simulink model "CS_PIDPr"  (R2014b)
settings: Solver=ode5  StartTime=0.0  StopTime=Te  FixedStep=Tm  RelTol=1e-3
StopFcn:
  | %salida(simout)
values from neighbouring files (symbols this model uses):
  D = 0    [globales.mat]
  I = 0    [globales.mat]
  Kb = 0    [globales.mat]
  P = 0.1    [globales.mat]
  Pf = 50    [globales.mat]
  Pi = -50    [globales.mat]
  Tm = 0.5    [globales.mat]
  Tp = 5    [globales.mat]
undefined symbols (not defined in the file or in its folder): A, B
undefined symbols (not defined in the file): Fcd, Fcp, Np
settings Model: ExtModeTrigDuration=100000  Creator=Equipo-Servo  LastModifiedBy=E. Rubio
settings DebuggingCC: UnderspecifiedInitializationDetection=Classic  MergeDetectMultiDrivingBlocksExec=none  StateNameClashWarn=warning
settings HardwareCC: ProdIntDivRoundTo=Zero  ProdEndianess=LittleEndian  ProdHWDeviceType=Generic->32-bit x86 compatible
settings RTWCC: SystemTargetFile=rtwin.tlc  TemplateMakefile=rtwin.tmf  Description=Real-Time Windows Target  ProcessScript=rtwin_make_rtw_hook  RTWCompilerOptimization=On
settings CodeAppCC: MaxIdLength=95
settings RTWinTargetCC: TargetLibSuffix=_rtwin.lib  TargetPreCompLibLocation=C:\Program Files\MATLAB\R2014b\toolbox\rtw\targets\rtwin\lib\win64

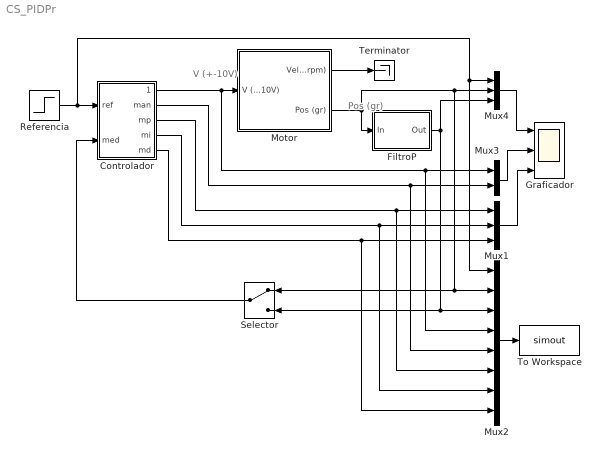
== system CS_PIDPr ==
  note: Pos
      | (gr)
  note: V (+-10V)
  Controlador : Subsystem  mask{T=Tm, P=P, I=I, Kb=Kb, D=D, Fcd=Fcd}
      mask prompts: T "Período de muestreo"; Kb "Kb (anti windup)"; Fcd "Fcd (Hz)"
      mask init:
      | N = 2*pi*Fcd;
  FiltroP : Subsystem  mask{N=Np, Fc=Fcp, Fm=1/Tm}
      mask prompts: N "Orden del filtro (Butterworth)"; Fc "Frecuencia de corte (Fc<Fm/2)"; Fm "Frecuencia de muestreo"
      mask init:
      | Fn = Fm/2;   % Frecuencia de Nyquist
      | [B,A] = butter(N,Fc/Fn);
  Graficador : Scope  NumInputPorts=3
      settings: TimeRange=10  YMin=-100~-15~-15  YMax=150~15~10  SampleTime=Tm
  Motor : Subsystem
  Mux1 : Mux  Inputs=3
  Mux2 : Mux  Inputs=8
  Mux3 : Mux  Inputs=2
  Mux4 : Mux  Inputs=3
  Referencia : Step  Time=Tp  Before=Pi  After=Pf  SampleTime=0
  Selector : ManualSwitch
  Terminator : Terminator
  To Workspace : ToWorkspace  VariableName=simout  SaveFormat=Structure With Time  SampleTime=Tm
  wires:
  Mux4/1 -> Graficador/1
  Motor/2(Pos (gr)) -> FiltroP/1(In), Selector/1, Mux2/2, Mux4/2
  Referencia/1 -> Mux2/1, Mux4/1, Controlador/1(ref)
  Mux2/1 -> To Workspace/1
  Controlador/1(mans) -> Motor/1(V (+-10V)), Mux2/4, Mux3/1
  FiltroP/1(Out) -> Selector/2, Mux2/3, Mux4/3
  Controlador/2(man) -> Mux2/5, Mux3/2
  Controlador/3(mp) -> Mux1/1, Mux2/6
  Controlador/4(mi) -> Mux2/7, Mux1/2
  Controlador/5(md) -> Mux2/8, Mux1/3
  Selector/1 -> Controlador/2(med)
  Mux3/1 -> Graficador/2
  Mux1/1 -> Graficador/3
  Motor/1(Vel (rpm)) -> Terminator/1

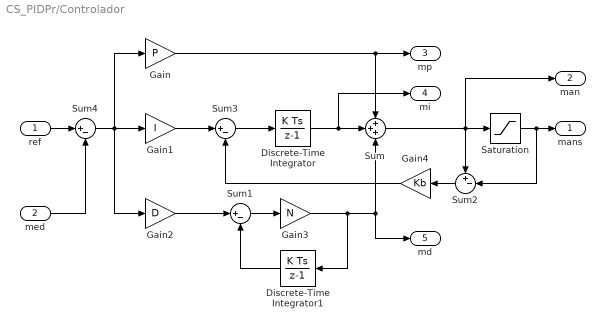
== system CS_PIDPr/Controlador ==
  ref : Inport
  med : Inport  Port=2
  Discrete-Time Integrator : DiscreteIntegrator  SampleTime=T
  Discrete-Time Integrator1 : DiscreteIntegrator  SampleTime=T
  Gain : Gain  Gain=P
  Gain1 : Gain  Gain=I
  Gain2 : Gain  Gain=D
  Gain3 : Gain  Gain=N
  Gain4 : Gain  Gain=Kb
  Saturation : Saturate  UpperLimit=10  LowerLimit=-10
  Sum : Sum  Inputs=+++
  Sum1 : Sum  Inputs=|+-
  Sum2 : Sum  Inputs=+-|
  Sum3 : Sum  Inputs=|+-
  Sum4 : Sum  Inputs=|+-
  mans : Outport
  man : Outport  Port=2
  mp : Outport  Port=3
  mi : Outport  Port=4
  md : Outport  Port=5
  wires:
  Sum/1 -> man/1, Sum2/1, Saturation/1
  Saturation/1 -> Sum2/2, mans/1
  Gain/1 -> Sum/1, mp/1
  Discrete-Time Integrator/1 -> mi/1, Sum/2
  ref/1 -> Sum4/1
  Sum1/1 -> Gain3/1
  Gain2/1 -> Sum1/1
  Discrete-Time Integrator1/1 -> Sum1/2
  Gain3/1 -> md/1, Sum/3, Discrete-Time Integrator1/1
  Sum2/1 -> Gain4/1
  Sum3/1 -> Discrete-Time Integrator/1
  Gain1/1 -> Sum3/1
  Gain4/1 -> Sum3/2
  Sum4/1 -> Gain2/1, Gain/1, Gain1/1
  med/1 -> Sum4/2

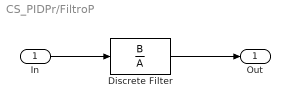
== system CS_PIDPr/FiltroP ==
  In : Inport
  Discrete Filter : DiscreteFilter  Numerator=B  Denominator=A  SampleTime=1/Fm
  Out : Outport
  wires:
  Discrete Filter/1 -> Out/1
  In/1 -> Discrete Filter/1

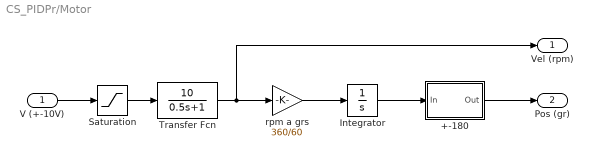
== system CS_PIDPr/Motor ==
  V (+-10V) : Inport
  +-180 : Subsystem
  Integrator : Integrator  InitialCondition=180  UpperSaturationLimit=180  LowerSaturationLimit=-180
  Saturation : Saturate  UpperLimit=10  LowerLimit=-10
  Transfer Fcn : TransferFcn  Numerator=[10]  Denominator=[0.5 1]
  rpm a grs : Gain  Gain=360/60
  Vel (rpm) : Outport
  Pos (gr) : Outport  Port=2
  wires:
  V (+-10V)/1 -> Saturation/1
  Transfer Fcn/1 -> Vel (rpm)/1, rpm a grs/1
  Integrator/1 -> +-180/1(In)
  Saturation/1 -> Transfer Fcn/1
  +-180/1(Out) -> Pos (gr)/1
  rpm a grs/1 -> Integrator/1

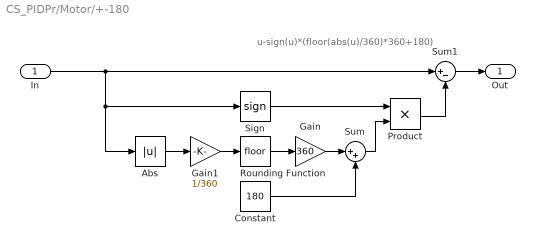
== system CS_PIDPr/Motor/+-180 ==
  note: u-sign(u)*(floor(abs(u)/360)*360+180)
  In : Inport
  Abs : Abs
  Constant : Constant  Value=180
  Gain : Gain  Gain=360
  Gain1 : Gain  Gain=1/360
  Product : Product
  Rounding Function : Rounding
  Sign : Signum
  Sum : Sum  Inputs=|++
  Sum1 : Sum  Inputs=|+-
  Out : Outport
  wires:
  Sum/1 -> Product/2
  Constant/1 -> Sum/2
  Sign/1 -> Product/1
  Gain1/1 -> Rounding Function/1
  Gain/1 -> Sum/1
  Rounding Function/1 -> Gain/1
  Sum1/1 -> Out/1
  Abs/1 -> Gain1/1
  Product/1 -> Sum1/2
  In/1 -> Abs/1, Sign/1, Sum1/1
